simulink model "CCModel_71"  (R2024a)
settings: Solver=ode3  StartTime=0.0  StopTime=100  FixedStep=0.001  RelTol=1e-3  EnableMultiTasking=on
undefined symbols (not defined in the file or in its folder): DiscIntNeverNeededParam, Hecate_desVel1, Hecate_desVel2, Hecate_desVel3, Hecate_horShift, Hecate_period, Hecate_slope, Hecate_Transition1, Hecate_Transition2, Hecate_verShift, i, PME_qb, qb_map, RPM_qb, V
libraries: simulink x46
(part 5 of 11)

== system CCModel_71/Cruise Control/Version 6.4/Sigmoid ==
  note: This whole part is just to eliminate weird cancellation errors that were happening
  U1 : Inport
  U2 : Inport  Port=2
  Change_time : Inport  Port=3
  Abs : Abs  SaturateOnIntegerOverflow=off
  Abs2 : Abs  SaturateOnIntegerOverflow=off
  Add Constant : Bias  Bias=1  SaturateOnIntegerOverflow=off
  Add Constant2 : Bias  Bias=1  SaturateOnIntegerOverflow=off
  Add Constant3 : Bias  Bias=1  SaturateOnIntegerOverflow=off
  Add3 : Sum
  Add4 : Sum  Inputs=+-
  Add5 : Sum
  Clock1 : Clock
  Constant : Constant
  Constant3 : Constant
  Divide : Product  Inputs=/*
  Divide1 : Product  Inputs=**
  Divide4 : Product  Inputs=*/
  Divide5 : Product  Inputs=**
  Divide6 : Product  Inputs=**
  Divide8 : Product  Inputs=*/
  Gain : Gain  Gain=1/2
  Gain1 : Gain  Gain=2
  Gain2 : Gain  Gain=1000
  Gain3 : Gain  Gain=0.001
  Gain5 : Gain  Gain=1/2
  K : Constant
  Power{,3..5} (4 alike) : Math  Operator=pow
  Reciprocal : Product  Inputs=/
  Reciprocal2 : Product  Inputs=/
  Round1 : Rounding  Operator=round
  Scope : Scope  NumInputPorts=3
  Subtract : Sum  Inputs=+-
  Subtract1 : Sum  Inputs=+-
  Subtract2 : Sum  Inputs=+-
  Sum1 : Sum  Inputs=|-+
  h : Constant  Value=4
  u_out : Outport
  wires:
  Add5/1 -> Scope/1, u_out/1
  h/1 -> Abs2/1, Divide8/1, Subtract/2
  Add3/1 -> Divide6/2
  Add4/1 -> Divide5/1
  Constant3/1 -> Add3/2, Add4/1
  Power5/1 -> Divide4/2
  Reciprocal2/1 -> Power5/2
  K/1 -> Power4/2, Reciprocal2/1, Reciprocal/1, Power/2
  Gain5/1 -> Divide6/1
  Change_time/1 -> Sum1/1
  Abs/1 -> Power4/1
  Clock1/1 -> Sum1/2
  Gain3/1 -> Subtract/1
  U2/1 -> Gain5/1, Scope/2, Divide1/1
  Round1/1 -> Gain3/1
  Power4/1 -> Add Constant/1
  Gain2/1 -> Round1/1
  Add Constant/1 -> Power5/1
  Subtract/1 -> Divide4/1, Abs/1
  U1/1 -> Subtract2/1, Scope/3
  Divide6/1 -> Add5/1
  Sum1/1 -> Gain2/1  "Elapsed Time"
  Divide4/1 -> Add3/1, Add4/2
  Abs2/1 -> Power/1
  Power/1 -> Add Constant2/1
  Add Constant2/1 -> Power3/1
  Reciprocal/1 -> Power3/2
  Power3/1 -> Divide8/2
  Divide8/1 -> Add Constant3/1
  Add Constant3/1 -> Gain/1
  Constant/1 -> Subtract1/1
  Gain/1 -> Gain1/1, Subtract1/2  "P"
  Subtract1/1 -> Divide1/2
  Divide1/1 -> Subtract2/2
  Subtract2/1 -> Divide/2
  Gain1/1 -> Divide/1
  Divide/1 -> Divide5/2
  Divide5/1 -> Add5/2

== system CCModel_71/Cruise Control/Version 6.4/Switches ==
  U : Inport
  Throttle_In : Inport  Port=2
  Brake_In : Inport  Port=3
  Brake_Switch1 : Switch  Criteria=u2 > Threshold  SaturateOnIntegerOverflow=off  InputSameDT=off
  Brake_Switch3 : Switch  Criteria=u2 > Threshold  Threshold=5  SaturateOnIntegerOverflow=off  InputSameDT=off
  Constant : Constant  Value=0
  Constant3 : Constant  Value=0
  Constant4 : Constant  Value=10
  Constant5 : Constant  Value=10
  Gain11 : Gain  Gain=0.9
  Gain13 : Gain  Gain=-1
  Gain8 : Gain  Gain=0.9
  Max1 : MinMax  Function=max  Inputs=2
  Plus2 : Sum
  Plus3 : Sum
  Polynomial : Polyval  Coefs=[-0.011, -0.12,0.9,10]
  Polynomial1 : Polyval  Coefs=[-0.011, -0.12,0.9,10]
  Ramp1 : simulink/Sources/Ramp  slope=1  start=0  InitialOutput=-100
  Saturation1 : Saturate  UpperLimit=100  LowerLimit=-100
  Scope1 : Scope  NumInputPorts=3
  Switch : Switch  Criteria=u2 > Threshold  Threshold=-10  SaturateOnIntegerOverflow=off  InputSameDT=off
  Switch1 : Switch  Criteria=u2 > Threshold  Threshold=10  SaturateOnIntegerOverflow=off  InputSameDT=off
  Throttle_Switch1 : Switch  Criteria=u2 > Threshold  SaturateOnIntegerOverflow=off  InputSameDT=off
  Throttle_Switch3 : Switch  Criteria=u2 > Threshold  Threshold=5  SaturateOnIntegerOverflow=off  InputSameDT=off
  Throttle : Outport
  Brake : Outport  Port=2
  wires:
  Plus2/1 -> Throttle_Switch1/1
  Gain8/1 -> Plus2/1
  Constant4/1 -> Plus2/2
  Gain13/1 -> Polynomial1/1, Gain11/1, Brake_Switch1/2
  Constant5/1 -> Plus3/2
  Brake_Switch1/1 -> Brake_Switch3/3  "Brake"
  Throttle_Switch1/1 -> Throttle_Switch3/3  "Throttle"
  Gain11/1 -> Plus3/1
  Brake_Switch3/1 -> Scope1/3, Brake/1
  Brake_In/1 -> Brake_Switch3/1, Max1/2
  Switch/1 -> Throttle_Switch1/3
  Throttle_In/1 -> Throttle_Switch3/1, Max1/1
  Saturation1/1 -> Switch/2, Switch1/2, Gain13/1, Gain8/1, Throttle_Switch1/2, Scope1/1, Polynomial/1
  Polynomial/1 -> Switch/1
  Polynomial1/1 -> Switch1/3
  Constant/1 -> Switch/3
  Switch1/1 -> Brake_Switch1/3
  Constant3/1 -> Switch1/1
  Throttle_Switch3/1 -> Scope1/2, Throttle/1
  Max1/1 -> Throttle_Switch3/2, Brake_Switch3/2
  Plus3/1 -> Brake_Switch1/1
  U/1 -> Saturation1/1

== system CCModel_71/Cruise Control/Version 6.5/Apply_Grade ==
  note: This has not been implemented but may be helpful
  note: +(2/5)|P|
  note: x is u, which is linear and g is grade which is sigmoided
  U_in : Inport
  Grade : Inport  Port=2
  Add : Sum
  Add Constant : Bias  Bias=1  SaturateOnIntegerOverflow=off
  Divide : Product  Inputs=*/
  Gain : Gain  Gain=0.8
  Gain1 : Gain  Gain=0.25
  Scope : Scope  NumInputPorts=2
  Sqrt : Sqrt
  Square : Math  Operator=square
  U_Out : Outport
  wires:
  U_in/1 -> Scope/1, Gain/1
  Square/1 -> Add Constant/1
  Add Constant/1 -> Sqrt/1
  Grade/1 -> Gain1/1, Square/1
  Gain1/1 -> Divide/1
  Sqrt/1 -> Divide/2
  Divide/1 -> Add/2
  Gain/1 -> Add/1
  Add/1 -> Scope/2, U_Out/1

== system CCModel_71/Cruise Control/Version 6.5/Detect Change ==
  note: This subsystem detects either a change in the reference velocity, or the driver releasing one of the pedals. It outputs the time of the change, the value of u just before the change, and a boolean "hasChanged" value
  desired_velocity : Inport
  throttle_const : Inport  Port=2
  brake_const : Inport  Port=3
  Smoothed u : Inport  Port=4
  (False) : Constant  Value=0
  (True) : Constant
  AND : Logic  IconShape=distinctive  AllPortsSameDT=off  OutDataTypeStr=boolean
  Clock : Clock
  Constant : Constant  Value=0.01
  Delay : Delay  DelayLength=1
  Delay1 : Delay  DelayLength=1
  Detect Change : simulink/Logic and Bit Operations/Detect Change  vinit=0  OutDataTypeStr=boolean
  Detect Change1 : simulink/Logic and Bit Operations/Detect Change  vinit=0  OutDataTypeStr=boolean
  Max : MinMax  Function=max  Inputs=2
  Max1 : MinMax  Function=max  Inputs=2
  OR : Logic  Operator=OR  IconShape=distinctive  AllPortsSameDT=off  OutDataTypeStr=boolean
  Pedal_threshold : Constant
  Scope : Scope
  Subtract : Sum  Inputs=+-
  Switch : Switch  Criteria=u2 > Threshold  SaturateOnIntegerOverflow=off  InputSameDT=off
  Switch1 : Switch  Criteria=u2 > Threshold  SaturateOnIntegerOverflow=off  InputSameDT=off
  Switch2 : Switch  Criteria=u2 > Threshold  SaturateOnIntegerOverflow=off  InputSameDT=off
  Change_time : Outport
  Old u : Outport  Port=2
  hasChanged : Outport  Port=3
  wires:
  desired_velocity/1 -> Detect Change/1
  Detect Change/1 -> OR/1
  OR/1 -> Switch/2, Switch2/2, hasChanged/1
  Switch1/1 -> Detect Change1/1, Delay1/1
  AND/1 -> OR/2
  Clock/1 -> Switch/1
  Max/1 -> Subtract/1
  (True)/1 -> Switch1/1
  brake_const/1 -> Max/2
  Pedal_threshold/1 -> Subtract/2
  Subtract/1 -> Switch1/2
  (False)/1 -> Switch1/3
  throttle_const/1 -> Max/1
  Switch2/1 -> Switch2/3, Max1/1
  Delay/1 -> Switch2/1
  Switch/1 -> Switch/3, Scope/1, Change_time/1
  Smoothed u/1 -> Delay/1
  Detect Change1/1 -> AND/2
  Delay1/1 -> AND/1
  Constant/1 -> Max1/2
  Max1/1 -> Old u/1

== system CCModel_71/Cruise Control/Version 6.5/PID Controller ==
  note: Typical PID controller, outputs a value between -100 and 100
  error : Inport
  Grade : Inport  Port=2
  Add : Sum
  Add1 : Sum
  Derivative : Derivative
  GKi : Gain  Gain=0
  GKp : Gain  Gain=0
  Integrator : Integrator
  Integrator1 : Integrator
  Kd : Gain  Gain=0.1
  Ki : Gain  Gain=0.03
  Kp : Gain  Gain=4
  Saturation : Saturate  UpperLimit=100  LowerLimit=-100
  Scope1 : Scope  NumInputPorts=3
  Sum : Sum  Inputs=+++
  u : Outport
  wires:
  Integrator/1 -> Ki/1
  error/1 -> Integrator/1, Kp/1, Derivative/1  "D"
  Kp/1 -> Scope1/1, Sum/2  "P"
  Ki/1 -> Sum/1, Scope1/2  "I"
  Saturation/1 -> u/1
  Derivative/1 -> Kd/1
  Kd/1 -> Scope1/3, Sum/3  "D"
  Sum/1 -> Add1/1
  Add1/1 -> Saturation/1
  Grade/1 -> Integrator1/1, GKp/1
  Integrator1/1 -> GKi/1
  GKi/1 -> Add/1
  GKp/1 -> Add/2
  Add/1 -> Add1/2

== system CCModel_71/Cruise Control/Version 6.5/Sigmoid ==
  note: This whole part is just to eliminate weird cancellation errors that were happening
  U1 : Inport
  U2 : Inport  Port=2
  Change_time : Inport  Port=3
  Abs : Abs  SaturateOnIntegerOverflow=off
  Abs2 : Abs  SaturateOnIntegerOverflow=off
  Add Constant : Bias  Bias=1  SaturateOnIntegerOverflow=off
  Add Constant2 : Bias  Bias=1  SaturateOnIntegerOverflow=off
  Add Constant3 : Bias  Bias=1  SaturateOnIntegerOverflow=off
  Add3 : Sum
  Add4 : Sum  Inputs=+-
  Add5 : Sum
  Clock1 : Clock
  Constant : Constant
  Constant3 : Constant
  Divide : Product  Inputs=/*
  Divide1 : Product  Inputs=**
  Divide4 : Product  Inputs=*/
  Divide5 : Product  Inputs=**
  Divide6 : Product  Inputs=**
  Divide8 : Product  Inputs=*/
  Gain : Gain  Gain=1/2
  Gain1 : Gain  Gain=2
  Gain2 : Gain  Gain=1000
  Gain3 : Gain  Gain=0.001
  Gain5 : Gain  Gain=1/2
  K : Constant  Value=1.5
  Power{,3..5} (4 alike) : Math  Operator=pow
  Reciprocal : Product  Inputs=/
  Reciprocal2 : Product  Inputs=/
  Round1 : Rounding  Operator=round
  Scope : Scope  NumInputPorts=3
  Subtract : Sum  Inputs=+-
  Subtract1 : Sum  Inputs=+-
  Subtract2 : Sum  Inputs=+-
  Sum1 : Sum  Inputs=|-+
  h : Constant  Value=4
  u_out : Outport
  wires:
  Add5/1 -> Scope/1, u_out/1
  h/1 -> Abs2/1, Divide8/1, Subtract/2
  Add3/1 -> Divide6/2
  Add4/1 -> Divide5/1
  Constant3/1 -> Add3/2, Add4/1
  Power5/1 -> Divide4/2
  Reciprocal2/1 -> Power5/2
  K/1 -> Power4/2, Reciprocal2/1, Reciprocal/1, Power/2
  Gain5/1 -> Divide6/1
  Change_time/1 -> Sum1/1
  Abs/1 -> Power4/1
  Clock1/1 -> Sum1/2
  Gain3/1 -> Subtract/1
  U2/1 -> Gain5/1, Scope/2, Divide1/1
  Round1/1 -> Gain3/1
  Power4/1 -> Add Constant/1
  Gain2/1 -> Round1/1
  Add Constant/1 -> Power5/1
  Subtract/1 -> Divide4/1, Abs/1
  U1/1 -> Subtract2/1, Scope/3
  Divide6/1 -> Add5/1
  Sum1/1 -> Gain2/1  "Elapsed Time"
  Divide4/1 -> Add3/1, Add4/2
  Abs2/1 -> Power/1
  Power/1 -> Add Constant2/1
  Add Constant2/1 -> Power3/1
  Reciprocal/1 -> Power3/2
  Power3/1 -> Divide8/2
  Divide8/1 -> Add Constant3/1
  Add Constant3/1 -> Gain/1
  Constant/1 -> Subtract1/1
  Gain/1 -> Gain1/1, Subtract1/2  "P"
  Subtract1/1 -> Divide1/2
  Divide1/1 -> Subtract2/2
  Subtract2/1 -> Divide/2
  Gain1/1 -> Divide/1
  Divide/1 -> Divide5/2
  Divide5/1 -> Add5/2

== system CCModel_71/Cruise Control/Version 6.5/Switches ==
  U : Inport
  Throttle_In : Inport  Port=2
  Brake_In : Inport  Port=3
  Brake_Switch1 : Switch  Criteria=u2 > Threshold  SaturateOnIntegerOverflow=off  InputSameDT=off
  Brake_Switch3 : Switch  Criteria=u2 > Threshold  Threshold=5  SaturateOnIntegerOverflow=off  InputSameDT=off
  Constant : Constant  Value=0
  Constant1 : Constant  Value=0
  Gain13 : Gain  Gain=-1
  Max1 : MinMax  Function=max  Inputs=2
  Polynomial : Polyval  Coefs=[-0.01,0.2,0,0]
  Polynomial1 : Polyval  Coefs=[-0.01,0.2,0,0]
  Ramp1 : simulink/Sources/Ramp  slope=5  start=0  InitialOutput=-100
  Saturation1 : Saturate  UpperLimit=100  LowerLimit=-100
  Scope1 : Scope  NumInputPorts=3
  Switch : Switch  Criteria=u2 > Threshold  Threshold=10  SaturateOnIntegerOverflow=off  InputSameDT=off
  Switch1 : Switch  Criteria=u2 > Threshold  Threshold=10  SaturateOnIntegerOverflow=off  InputSameDT=off
  Throttle_Switch1 : Switch  Criteria=u2 > Threshold  SaturateOnIntegerOverflow=off  InputSameDT=off
  Throttle_Switch3 : Switch  Criteria=u2 > Threshold  Threshold=5  SaturateOnIntegerOverflow=off  InputSameDT=off
  Throttle : Outport
  Brake : Outport  Port=2
  wires:
  Gain13/1 -> Polynomial1/1, Switch1/2, Switch1/1, Brake_Switch1/2
  Brake_Switch1/1 -> Brake_Switch3/3  "Brake"
  Throttle_Switch1/1 -> Throttle_Switch3/3  "Throttle"
  Brake_Switch3/1 -> Scope1/3, Brake/1
  Brake_In/1 -> Brake_Switch3/1, Max1/2
  Throttle_In/1 -> Throttle_Switch3/1, Max1/1
  Polynomial1/1 -> Switch1/3
  Throttle_Switch3/1 -> Scope1/2, Throttle/1
  Constant1/1 -> Brake_Switch1/3, Throttle_Switch1/3
  Switch/1 -> Throttle_Switch1/1
  Polynomial/1 -> Switch/3
  Switch1/1 -> Brake_Switch1/1
  Saturation1/1 -> Gain13/1, Switch/1, Switch/2, Scope1/1, Polynomial/1, Throttle_Switch1/2
  U/1 -> Saturation1/1
  Max1/1 -> Throttle_Switch3/2, Brake_Switch3/2

== system CCModel_71/Cruise Control/Version 6.6/Apply_Grade ==
  note: This has not been implemented but may be helpful
  note: +(2/5)|P|
  note: x is u, which is linear and g is grade which is sigmoided
  U_in : Inport
  Grade : Inport  Port=2
  Add : Sum
  Add Constant : Bias  Bias=1  SaturateOnIntegerOverflow=off
  Divide : Product  Inputs=*/
  Gain : Gain  Gain=0.8
  Gain1 : Gain  Gain=0.25
  Scope : Scope  NumInputPorts=2
  Sqrt : Sqrt
  Square : Math  Operator=square
  U_Out : Outport
  wires:
  U_in/1 -> Scope/1, Gain/1
  Square/1 -> Add Constant/1
  Add Constant/1 -> Sqrt/1
  Grade/1 -> Gain1/1, Square/1
  Gain1/1 -> Divide/1
  Sqrt/1 -> Divide/2
  Divide/1 -> Add/2
  Gain/1 -> Add/1
  Add/1 -> Scope/2, U_Out/1

== system CCModel_71/Cruise Control/Version 6.6/Detect Change ==
  note: This subsystem detects either a change in the reference velocity, or the driver releasing one of the pedals. It outputs the time of the change, the value of u just before the change, and a boolean "hasChanged" value
  desired_velocity : Inport
  throttle_const : Inport  Port=2
  brake_const : Inport  Port=3
  Smoothed u : Inport  Port=4
  (False) : Constant  Value=0
  (True) : Constant
  AND : Logic  IconShape=distinctive  AllPortsSameDT=off  OutDataTypeStr=boolean
  Clock : Clock
  Constant : Constant  Value=0.01
  Delay : Delay  DelayLength=1
  Delay1 : Delay  DelayLength=1
  Detect Change : simulink/Logic and Bit Operations/Detect Change  vinit=0  OutDataTypeStr=boolean
  Detect Change1 : simulink/Logic and Bit Operations/Detect Change  vinit=0  OutDataTypeStr=boolean
  Max : MinMax  Function=max  Inputs=2
  Max1 : MinMax  Function=max  Inputs=2
  OR : Logic  Operator=OR  IconShape=distinctive  AllPortsSameDT=off  OutDataTypeStr=boolean
  Pedal_threshold : Constant
  Scope : Scope
  Subtract : Sum  Inputs=+-
  Switch : Switch  Criteria=u2 > Threshold  SaturateOnIntegerOverflow=off  InputSameDT=off
  Switch1 : Switch  Criteria=u2 > Threshold  SaturateOnIntegerOverflow=off  InputSameDT=off
  Switch2 : Switch  Criteria=u2 > Threshold  SaturateOnIntegerOverflow=off  InputSameDT=off
  Change_time : Outport
  Old u : Outport  Port=2
  hasChanged : Outport  Port=3
  wires:
  desired_velocity/1 -> Detect Change/1
  Detect Change/1 -> OR/1
  OR/1 -> Switch/2, Switch2/2, hasChanged/1
  Switch1/1 -> Detect Change1/1, Delay1/1
  AND/1 -> OR/2
  Clock/1 -> Switch/1
  Max/1 -> Subtract/1
  (True)/1 -> Switch1/1
  brake_const/1 -> Max/2
  Pedal_threshold/1 -> Subtract/2
  Subtract/1 -> Switch1/2
  (False)/1 -> Switch1/3
  throttle_const/1 -> Max/1
  Switch2/1 -> Switch2/3, Max1/1
  Delay/1 -> Switch2/1
  Switch/1 -> Switch/3, Scope/1, Change_time/1
  Smoothed u/1 -> Delay/1
  Detect Change1/1 -> AND/2
  Delay1/1 -> AND/1
  Constant/1 -> Max1/2
  Max1/1 -> Old u/1

== system CCModel_71/Cruise Control/Version 6.6/PID Controller ==
  note: Typical PID controller, outputs a value between -100 and 100
  error : Inport
  Grade : Inport  Port=2
  Add : Sum
  Add1 : Sum
  Derivative : Derivative
  GKi : Gain  Gain=0
  GKp : Gain  Gain=0
  Integrator : Integrator
  Integrator1 : Integrator
  Kd : Gain  Gain=0.1
  Ki : Gain  Gain=0.03
  Kp : Gain  Gain=3
  Saturation : Saturate  Commented=through  UpperLimit=100  LowerLimit=-100
  Scope1 : Scope  NumInputPorts=3
  Sum : Sum  Inputs=+++
  u : Outport
  wires:
  Integrator/1 -> Ki/1
  error/1 -> Integrator/1, Kp/1, Derivative/1  "D"
  Kp/1 -> Scope1/1, Sum/2  "P"
  Ki/1 -> Sum/1, Scope1/2  "I"
  Saturation/1 -> u/1
  Derivative/1 -> Kd/1
  Kd/1 -> Scope1/3, Sum/3  "D"
  Sum/1 -> Add1/1
  Add1/1 -> Saturation/1
  Grade/1 -> Integrator1/1, GKp/1
  Integrator1/1 -> GKi/1
  GKi/1 -> Add/1
  GKp/1 -> Add/2
  Add/1 -> Add1/2

== system CCModel_71/Cruise Control/Version 6.6/Sigmoid ==
  note: This whole part is just to eliminate weird cancellation errors that were happening
  U1 : Inport
  U2 : Inport  Port=2
  Change_time : Inport  Port=3
  Abs : Abs  SaturateOnIntegerOverflow=off
  Abs2 : Abs  SaturateOnIntegerOverflow=off
  Add Constant : Bias  Bias=1  SaturateOnIntegerOverflow=off
  Add Constant2 : Bias  Bias=1  SaturateOnIntegerOverflow=off
  Add Constant3 : Bias  Bias=1  SaturateOnIntegerOverflow=off
  Add3 : Sum
  Add4 : Sum  Inputs=+-
  Add5 : Sum
  Clock1 : Clock
  Constant : Constant
  Constant3 : Constant
  Divide : Product  Inputs=/*
  Divide1 : Product  Inputs=**
  Divide4 : Product  Inputs=*/
  Divide5 : Product  Inputs=**
  Divide6 : Product  Inputs=**
  Divide8 : Product  Inputs=*/
  Gain : Gain  Gain=1/2
  Gain1 : Gain  Gain=2
  Gain2 : Gain  Gain=1000
  Gain3 : Gain  Gain=0.001
  Gain5 : Gain  Gain=1/2
  K : Constant  Value=1.5
  Power{,3..5} (4 alike) : Math  Operator=pow
  Reciprocal : Product  Inputs=/
  Reciprocal2 : Product  Inputs=/
  Round1 : Rounding  Operator=round
  Saturation : Saturate  UpperLimit=100  LowerLimit=-100
  Scope : Scope  NumInputPorts=3
  Subtract : Sum  Inputs=+-
  Subtract1 : Sum  Inputs=+-
  Subtract2 : Sum  Inputs=+-
  Sum1 : Sum  Inputs=|-+
  h : Constant  Value=4
  u_out : Outport
  wires:
  Add5/1 -> Scope/1, Saturation/1
  h/1 -> Abs2/1, Divide8/1, Subtract/2
  Add3/1 -> Divide6/2
  Add4/1 -> Divide5/1
  Constant3/1 -> Add3/2, Add4/1
  Power5/1 -> Divide4/2
  Reciprocal2/1 -> Power5/2
  K/1 -> Power4/2, Reciprocal2/1, Reciprocal/1, Power/2
  Gain5/1 -> Divide6/1
  Change_time/1 -> Sum1/1
  Abs/1 -> Power4/1
  Clock1/1 -> Sum1/2
  Gain3/1 -> Subtract/1
  U2/1 -> Gain5/1, Scope/2, Divide1/1
  Round1/1 -> Gain3/1
  Power4/1 -> Add Constant/1
  Gain2/1 -> Round1/1
  Add Constant/1 -> Power5/1
  Subtract/1 -> Divide4/1, Abs/1
  U1/1 -> Subtract2/1, Scope/3
  Divide6/1 -> Add5/1
  Sum1/1 -> Gain2/1  "Elapsed Time"
  Divide4/1 -> Add3/1, Add4/2
  Abs2/1 -> Power/1
  Power/1 -> Add Constant2/1
  Add Constant2/1 -> Power3/1
  Reciprocal/1 -> Power3/2
  Power3/1 -> Divide8/2
  Divide8/1 -> Add Constant3/1
  Add Constant3/1 -> Gain/1
  Constant/1 -> Subtract1/1
  Gain/1 -> Gain1/1, Subtract1/2  "P"
  Subtract1/1 -> Divide1/2
  Divide1/1 -> Subtract2/2
  Subtract2/1 -> Divide/2
  Gain1/1 -> Divide/1
  Divide/1 -> Divide5/2
  Divide5/1 -> Add5/2
  Saturation/1 -> u_out/1

== system CCModel_71/Cruise Control/Version 6.6/Switches ==
  U : Inport
  Throttle_In : Inport  Port=2
  Brake_In : Inport  Port=3
  Brake_Switch1 : Switch  Criteria=u2 > Threshold  SaturateOnIntegerOverflow=off  InputSameDT=off
  Brake_Switch3 : Switch  Criteria=u2 > Threshold  Threshold=5  SaturateOnIntegerOverflow=off  InputSameDT=off
  Constant : Constant  Value=0
  Constant1 : Constant  Value=0
  Gain13 : Gain  Gain=-1
  Max1 : MinMax  Function=max  Inputs=2
  Polynomial : Polyval  Coefs=[-0.01,0.2,0,0]
  Polynomial1 : Polyval  Coefs=[-0.01,0.2,0,0]
  Ramp1 : simulink/Sources/Ramp  slope=5  start=0  InitialOutput=-100
  Saturation1 : Saturate  UpperLimit=100  LowerLimit=-100
  Scope1 : Scope  NumInputPorts=3
  Switch : Switch  Criteria=u2 > Threshold  Threshold=10  SaturateOnIntegerOverflow=off  InputSameDT=off
  Switch1 : Switch  Criteria=u2 > Threshold  Threshold=10  SaturateOnIntegerOverflow=off  InputSameDT=off
  Throttle_Switch1 : Switch  Criteria=u2 > Threshold  SaturateOnIntegerOverflow=off  InputSameDT=off
  Throttle_Switch3 : Switch  Criteria=u2 > Threshold  Threshold=5  SaturateOnIntegerOverflow=off  InputSameDT=off
  Throttle : Outport
  Brake : Outport  Port=2
  wires:
  Gain13/1 -> Polynomial1/1, Switch1/2, Switch1/1, Brake_Switch1/2
  Brake_Switch1/1 -> Brake_Switch3/3  "Brake"
  Throttle_Switch1/1 -> Throttle_Switch3/3  "Throttle"
  Brake_Switch3/1 -> Scope1/3, Brake/1
  Brake_In/1 -> Brake_Switch3/1, Max1/2
  Throttle_In/1 -> Throttle_Switch3/1, Max1/1
  Polynomial1/1 -> Switch1/3
  Throttle_Switch3/1 -> Scope1/2, Throttle/1
  Constant1/1 -> Brake_Switch1/3, Throttle_Switch1/3
  Switch/1 -> Throttle_Switch1/1
  Polynomial/1 -> Switch/3
  Switch1/1 -> Brake_Switch1/1
  Saturation1/1 -> Gain13/1, Switch/1, Switch/2, Scope1/1, Polynomial/1, Throttle_Switch1/2
  U/1 -> Saturation1/1
  Max1/1 -> Throttle_Switch3/2, Brake_Switch3/2

== system CCModel_71/Cruise Control/Version 7.0/Apply_Grade ==
  note: This has not been implemented but may be helpful
  note: +(2/5)|P|
  note: x is u, which is linear and g is grade which is sigmoided
  U_in : Inport
  Grade : Inport  Port=2
  Add : Sum
  Add Constant : Bias  Bias=1  SaturateOnIntegerOverflow=off
  Divide : Product  Inputs=*/
  Gain : Gain  Gain=0.8
  Gain1 : Gain  Gain=0.25
  Scope : Scope  NumInputPorts=2
  Sqrt : Sqrt
  Square : Math  Operator=square
  U_Out : Outport
  wires:
  U_in/1 -> Scope/1, Gain/1
  Square/1 -> Add Constant/1
  Add Constant/1 -> Sqrt/1
  Grade/1 -> Gain1/1, Square/1
  Gain1/1 -> Divide/1
  Sqrt/1 -> Divide/2
  Divide/1 -> Add/2
  Gain/1 -> Add/1
  Add/1 -> Scope/2, U_Out/1

== system CCModel_71/Cruise Control/Version 7.0/Detect Change ==
  note: This subsystem detects either a change in the reference velocity, or the driver releasing one of the pedals. It outputs the time of the change, the value of u just before the change, and a boolean "hasChanged" value
  desired_velocity : Inport
  throttle_const : Inport  Port=2
  brake_const : Inport  Port=3
  Smoothed u : Inport  Port=4
  (False) : Constant  Value=0
  (True) : Constant
  AND : Logic  IconShape=distinctive  AllPortsSameDT=off  OutDataTypeStr=boolean
  Clock : Clock
  Constant : Constant  Value=0.01
  Delay : Delay  DelayLength=1
  Delay1 : Delay  DelayLength=1
  Detect Change : simulink/Logic and Bit Operations/Detect Change  vinit=0  OutDataTypeStr=boolean
  Detect Change1 : simulink/Logic and Bit Operations/Detect Change  vinit=0  OutDataTypeStr=boolean
  Max : MinMax  Function=max  Inputs=2
  Max1 : MinMax  Function=max  Inputs=2
  OR : Logic  Operator=OR  IconShape=distinctive  AllPortsSameDT=off  OutDataTypeStr=boolean
  Pedal_threshold : Constant
  Scope : Scope
  Subtract : Sum  Inputs=+-
  Switch : Switch  Criteria=u2 > Threshold  SaturateOnIntegerOverflow=off  InputSameDT=off
  Switch1 : Switch  Criteria=u2 > Threshold  SaturateOnIntegerOverflow=off  InputSameDT=off
  Switch2 : Switch  Criteria=u2 > Threshold  SaturateOnIntegerOverflow=off  InputSameDT=off
  Change_time : Outport
  Old u : Outport  Port=2
  hasChanged : Outport  Port=3
  wires:
  desired_velocity/1 -> Detect Change/1
  Detect Change/1 -> OR/1
  OR/1 -> Switch/2, Switch2/2, hasChanged/1
  Switch1/1 -> Detect Change1/1, Delay1/1
  AND/1 -> OR/2
  Clock/1 -> Switch/1
  Max/1 -> Subtract/1
  (True)/1 -> Switch1/1
  brake_const/1 -> Max/2
  Pedal_threshold/1 -> Subtract/2
  Subtract/1 -> Switch1/2
  (False)/1 -> Switch1/3
  throttle_const/1 -> Max/1
  Switch2/1 -> Switch2/3, Max1/1
  Delay/1 -> Switch2/1
  Switch/1 -> Switch/3, Scope/1, Change_time/1
  Smoothed u/1 -> Delay/1
  Detect Change1/1 -> AND/2
  Delay1/1 -> AND/1
  Constant/1 -> Max1/2
  Max1/1 -> Old u/1

== system CCModel_71/Cruise Control/Version 7.0/PID Controller ==
  note: Typical PID controller, outputs a value between -100 and 100
  error : Inport
  Grade : Inport  Port=2
  Add : Sum
  Add1 : Sum
  Derivative : Derivative
  GKi : Gain  Gain=0
  GKp : Gain  Gain=0
  Integrator : Integrator
  Integrator1 : Integrator
  Kd : Gain  Gain=0.1
  Ki : Gain  Gain=0.03
  Kp : Gain  Gain=4
  Saturation : Saturate  Commented=through  UpperLimit=100  LowerLimit=-100
  Scope1 : Scope  NumInputPorts=3
  Sum : Sum  Inputs=+++
  u : Outport
  wires:
  Integrator/1 -> Ki/1
  error/1 -> Integrator/1, Kp/1, Derivative/1  "D"
  Kp/1 -> Scope1/1, Sum/2  "P"
  Ki/1 -> Sum/1, Scope1/2  "I"
  Saturation/1 -> u/1
  Derivative/1 -> Kd/1
  Kd/1 -> Scope1/3, Sum/3  "D"
  Sum/1 -> Add1/1
  Add1/1 -> Saturation/1
  Grade/1 -> Integrator1/1, GKp/1
  Integrator1/1 -> GKi/1
  GKi/1 -> Add/1
  GKp/1 -> Add/2
  Add/1 -> Add1/2

== system CCModel_71/Cruise Control/Version 7.0/Sigmoid ==
  note: This whole part is just to eliminate weird cancellation errors that were happening
  U1 : Inport
  U2 : Inport  Port=2
  Change_time : Inport  Port=3
  Abs : Abs  SaturateOnIntegerOverflow=off
  Abs2 : Abs  SaturateOnIntegerOverflow=off
  Add Constant : Bias  Bias=1  SaturateOnIntegerOverflow=off
  Add Constant2 : Bias  Bias=1  SaturateOnIntegerOverflow=off
  Add Constant3 : Bias  Bias=1  SaturateOnIntegerOverflow=off
  Add3 : Sum
  Add4 : Sum  Inputs=+-
  Add5 : Sum
  Clock1 : Clock
  Constant : Constant
  Constant3 : Constant
  Divide : Product  Inputs=/*
  Divide1 : Product  Inputs=**
  Divide4 : Product  Inputs=*/
  Divide5 : Product  Inputs=**
  Divide6 : Product  Inputs=**
  Divide8 : Product  Inputs=*/
  Gain : Gain  Gain=1/2
  Gain1 : Gain  Gain=2
  Gain2 : Gain  Gain=1000
  Gain3 : Gain  Gain=0.001
  Gain5 : Gain  Gain=1/2
  K : Constant  Value=1.5
  Power{,3..5} (4 alike) : Math  Operator=pow
  Reciprocal : Product  Inputs=/
  Reciprocal2 : Product  Inputs=/
  Round1 : Rounding  Operator=round
  Saturation : Saturate  UpperLimit=100  LowerLimit=-100
  Scope : Scope  NumInputPorts=3
  Subtract : Sum  Inputs=+-
  Subtract1 : Sum  Inputs=+-
  Subtract2 : Sum  Inputs=+-
  Sum1 : Sum  Inputs=|-+
  h : Constant  Value=4
  u_out : Outport
  wires:
  Add5/1 -> Scope/1, Saturation/1
  h/1 -> Abs2/1, Divide8/1, Subtract/2
  Add3/1 -> Divide6/2
  Add4/1 -> Divide5/1
  Constant3/1 -> Add3/2, Add4/1
  Power5/1 -> Divide4/2
  Reciprocal2/1 -> Power5/2
  K/1 -> Power4/2, Reciprocal2/1, Reciprocal/1, Power/2
  Gain5/1 -> Divide6/1
  Change_time/1 -> Sum1/1
  Abs/1 -> Power4/1
  Clock1/1 -> Sum1/2
  Gain3/1 -> Subtract/1
  U2/1 -> Gain5/1, Scope/2, Divide1/1
  Round1/1 -> Gain3/1
  Power4/1 -> Add Constant/1
  Gain2/1 -> Round1/1
  Add Constant/1 -> Power5/1
  Subtract/1 -> Divide4/1, Abs/1
  U1/1 -> Subtract2/1, Scope/3
  Divide6/1 -> Add5/1
  Sum1/1 -> Gain2/1  "Elapsed Time"
  Divide4/1 -> Add3/1, Add4/2
  Abs2/1 -> Power/1
  Power/1 -> Add Constant2/1
  Add Constant2/1 -> Power3/1
  Reciprocal/1 -> Power3/2
  Power3/1 -> Divide8/2
  Divide8/1 -> Add Constant3/1
  Add Constant3/1 -> Gain/1
  Constant/1 -> Subtract1/1
  Gain/1 -> Gain1/1, Subtract1/2  "P"
  Subtract1/1 -> Divide1/2
  Divide1/1 -> Subtract2/2
  Subtract2/1 -> Divide/2
  Gain1/1 -> Divide/1
  Divide/1 -> Divide5/2
  Divide5/1 -> Add5/2
  Saturation/1 -> u_out/1

== system CCModel_71/Cruise Control/Version 7.0/Switches ==
  U : Inport
  Throttle_In : Inport  Port=2
  Brake_In : Inport  Port=3
  Add Constant : Bias  Bias=6  SaturateOnIntegerOverflow=off
  Add Constant1 : Bias  Bias=10  SaturateOnIntegerOverflow=off
  Add Constant2 : Bias  Bias=5  SaturateOnIntegerOverflow=off
  Add Constant3 : Bias  Bias=-10  SaturateOnIntegerOverflow=off
  Brake_Switch1 : Switch  Criteria=u2 > Threshold  Threshold=-10  SaturateOnIntegerOverflow=off  InputSameDT=off
  Brake_Switch2 : Switch  Criteria=u2 > Threshold  Threshold=30  SaturateOnIntegerOverflow=off  InputSameDT=off
  Brake_Switch3 : Switch  Criteria=u2 > Threshold  Threshold=5  SaturateOnIntegerOverflow=off  InputSameDT=off
  Constant : Constant  Value=0
  Constant1 : Constant  Value=0
  Gain : Gain  Gain=-1
  Gain1 : Gain  Gain=pi/40
  Gain2 : Gain  Gain=-5
  Gain3 : Gain  Gain=0.2
  Max1 : MinMax  Function=max  Inputs=2
  Polynomial : Polyval  Coefs=[-0.01,0.2,0,0]
  Polynomial1 : Polyval  Coefs=[0.01,0.2,0,10]
  Ramp1 : simulink/Sources/Ramp  slope=5  start=0  InitialOutput=-100
  Saturation1 : Saturate  UpperLimit=100  LowerLimit=-100
  Scope1 : Scope  NumInputPorts=3
  Sin : Trigonometry
  Switch : Switch  Criteria=u2 > Threshold  Threshold=10  SaturateOnIntegerOverflow=off  InputSameDT=off
  Switch1 : Switch  Criteria=u2 > Threshold  Threshold=-20  SaturateOnIntegerOverflow=off  InputSameDT=off
  Throttle_Switch1 : Switch  Criteria=u2 > Threshold  SaturateOnIntegerOverflow=off  InputSameDT=off
  Throttle_Switch3 : Switch  Criteria=u2 > Threshold  Threshold=5  SaturateOnIntegerOverflow=off  InputSameDT=off
  Throttle : Outport
  Brake : Outport  Port=2
  wires:
  Saturation1/1 -> Brake_Switch2/2, Brake_Switch1/2, Switch1/2, Gain/1, Add Constant3/1, Add Constant1/1, Switch/1, Switch/2, Scope1/1, Polynomial/1, Throttle_Switch1/2
  Throttle_Switch1/1 -> Add Constant/1  "Throttle"
  Brake_Switch3/1 -> Scope1/3, Brake/1
  Brake_In/1 -> Brake_Switch3/1, Max1/2
  Throttle_In/1 -> Throttle_Switch3/1, Max1/1
  Throttle_Switch3/1 -> Scope1/2, Throttle/1
  Constant1/1 -> Throttle_Switch1/3, Brake_Switch2/1
  Switch/1 -> Throttle_Switch1/1
  Polynomial/1 -> Switch/3
  Max1/1 -> Throttle_Switch3/2, Brake_Switch3/2
  Add Constant/1 -> Throttle_Switch3/3
  Add Constant1/1 -> Polynomial1/1
  Gain/1 -> Switch1/3
  Polynomial1/1 -> Switch1/1
  Switch1/1 -> Brake_Switch1/3
  Gain1/1 -> Sin/1
  Sin/1 -> Gain2/1
  Gain2/1 -> Add Constant2/1
  Add Constant2/1 -> Brake_Switch1/1
  Brake_Switch2/1 -> Gain3/1  "Brake"
  Brake_Switch1/1 -> Brake_Switch2/3  "Brake"
  U/1 -> Saturation1/1
  Add Constant3/1 -> Gain1/1
  Gain3/1 -> Brake_Switch3/3

== system CCModel_71/Cruise Control/Version 7.1/Apply_Grade ==
  note: This has not been implemented but may be helpful
  note: +(2/5)|P|
  note: x is u, which is linear and g is grade which is sigmoided
  U_in : Inport
  Grade : Inport  Port=2
  Add : Sum
  Add Constant : Bias  Bias=1  SaturateOnIntegerOverflow=off
  Divide : Product  Inputs=*/
  Gain : Gain  Gain=0.8
  Gain1 : Gain  Gain=0.25
  Scope : Scope  NumInputPorts=2
  Sqrt : Sqrt
  Square : Math  Operator=square
  U_Out : Outport
  wires:
  U_in/1 -> Scope/1, Gain/1
  Square/1 -> Add Constant/1
  Add Constant/1 -> Sqrt/1
  Grade/1 -> Gain1/1, Square/1
  Gain1/1 -> Divide/1
  Sqrt/1 -> Divide/2
  Divide/1 -> Add/2
  Gain/1 -> Add/1
  Add/1 -> Scope/2, U_Out/1

== system CCModel_71/Cruise Control/Version 7.1/Detect Change ==
  note: This subsystem detects either a change in the reference velocity, or the driver releasing one of the pedals. It outputs the time of the change, the value of u just before the change, and a boolean "hasChanged" value
  desired_velocity : Inport
  throttle_const : Inport  Port=2
  brake_const : Inport  Port=3
  Smoothed u : Inport  Port=4
  (False) : Constant  Value=0
  (True) : Constant
  AND : Logic  IconShape=distinctive  AllPortsSameDT=off  OutDataTypeStr=boolean
  Clock : Clock
  Constant : Constant  Value=0.01
  Delay : Delay  DelayLength=1
  Delay1 : Delay  DelayLength=1
  Detect Change : simulink/Logic and Bit Operations/Detect Change  vinit=0  OutDataTypeStr=boolean
  Detect Change1 : simulink/Logic and Bit Operations/Detect Change  vinit=0  OutDataTypeStr=boolean
  Max : MinMax  Function=max  Inputs=2
  Max1 : MinMax  Function=max  Inputs=2
  OR : Logic  Operator=OR  IconShape=distinctive  AllPortsSameDT=off  OutDataTypeStr=boolean
  Pedal_threshold : Constant
  Scope : Scope
  Subtract : Sum  Inputs=+-
  Switch : Switch  Criteria=u2 > Threshold  SaturateOnIntegerOverflow=off  InputSameDT=off
  Switch1 : Switch  Criteria=u2 > Threshold  SaturateOnIntegerOverflow=off  InputSameDT=off
  Switch2 : Switch  Criteria=u2 > Threshold  SaturateOnIntegerOverflow=off  InputSameDT=off
  Change_time : Outport
  Old u : Outport  Port=2
  hasChanged : Outport  Port=3
  wires:
  desired_velocity/1 -> Detect Change/1
  Detect Change/1 -> OR/1
  OR/1 -> Switch/2, Switch2/2, hasChanged/1
  Switch1/1 -> Detect Change1/1, Delay1/1
  AND/1 -> OR/2
  Clock/1 -> Switch/1
  Max/1 -> Subtract/1
  (True)/1 -> Switch1/1
  brake_const/1 -> Max/2
  Pedal_threshold/1 -> Subtract/2
  Subtract/1 -> Switch1/2
  (False)/1 -> Switch1/3
  throttle_const/1 -> Max/1
  Switch2/1 -> Switch2/3, Max1/1
  Delay/1 -> Switch2/1
  Switch/1 -> Switch/3, Scope/1, Change_time/1
  Smoothed u/1 -> Delay/1
  Detect Change1/1 -> AND/2
  Delay1/1 -> AND/1
  Constant/1 -> Max1/2
  Max1/1 -> Old u/1

== system CCModel_71/Cruise Control/Version 7.1/PID Controller ==
  note: Typical PID controller, outputs a value between -100 and 100
  error : Inport
  Grade : Inport  Port=2
  Add : Sum
  Add1 : Sum
  Derivative : Derivative
  GKi : Gain  Gain=0
  GKp : Gain  Gain=0
  Integrator : Integrator
  Integrator1 : Integrator
  Kd : Gain  Gain=0.1
  Ki : Gain  Gain=0.03
  Kp : Gain  Gain=4
  Saturation : Saturate  Commented=through  UpperLimit=100  LowerLimit=-100
  Scope1 : Scope  NumInputPorts=3
  Sum : Sum  Inputs=+++
  u : Outport
  wires:
  Integrator/1 -> Ki/1
  error/1 -> Integrator/1, Kp/1, Derivative/1  "D"
  Kp/1 -> Scope1/1, Sum/2  "P"
  Ki/1 -> Sum/1, Scope1/2  "I"
  Saturation/1 -> u/1
  Derivative/1 -> Kd/1
  Kd/1 -> Scope1/3, Sum/3  "D"
  Sum/1 -> Add1/1
  Add1/1 -> Saturation/1
  Grade/1 -> Integrator1/1, GKp/1
  Integrator1/1 -> GKi/1
  GKi/1 -> Add/1
  GKp/1 -> Add/2
  Add/1 -> Add1/2

== system CCModel_71/Cruise Control/Version 7.1/Sigmoid ==
  note: This whole part is just to eliminate weird cancellation errors that were happening
  U1 : Inport
  U2 : Inport  Port=2
  Change_time : Inport  Port=3
  Abs : Abs  SaturateOnIntegerOverflow=off
  Abs2 : Abs  SaturateOnIntegerOverflow=off
  Add Constant : Bias  Bias=1  SaturateOnIntegerOverflow=off
  Add Constant2 : Bias  Bias=1  SaturateOnIntegerOverflow=off
  Add Constant3 : Bias  Bias=1  SaturateOnIntegerOverflow=off
  Add3 : Sum
  Add4 : Sum  Inputs=+-
  Add5 : Sum
  Clock1 : Clock
  Constant : Constant
  Constant3 : Constant
  Divide : Product  Inputs=/*
  Divide1 : Product  Inputs=**
  Divide4 : Product  Inputs=*/
  Divide5 : Product  Inputs=**
  Divide6 : Product  Inputs=**
  Divide8 : Product  Inputs=*/
  Gain : Gain  Gain=1/2
  Gain1 : Gain  Gain=2
  Gain2 : Gain  Gain=1000
  Gain3 : Gain  Gain=0.001
  Gain5 : Gain  Gain=1/2
  K : Constant  Value=1.5
  Power{,3..5} (4 alike) : Math  Operator=pow
  Reciprocal : Product  Inputs=/
  Reciprocal2 : Product  Inputs=/
  Round1 : Rounding  Operator=round
  Saturation : Saturate  UpperLimit=100  LowerLimit=-100
  Scope : Scope  NumInputPorts=3
  Subtract : Sum  Inputs=+-
  Subtract1 : Sum  Inputs=+-
  Subtract2 : Sum  Inputs=+-
  Sum1 : Sum  Inputs=|-+
  h : Constant  Value=4
  u_out : Outport
  wires:
  Add5/1 -> Scope/1, Saturation/1
  h/1 -> Abs2/1, Divide8/1, Subtract/2
  Add3/1 -> Divide6/2
  Add4/1 -> Divide5/1
  Constant3/1 -> Add3/2, Add4/1
  Power5/1 -> Divide4/2
  Reciprocal2/1 -> Power5/2
  K/1 -> Power4/2, Reciprocal2/1, Reciprocal/1, Power/2
  Gain5/1 -> Divide6/1
  Change_time/1 -> Sum1/1
  Abs/1 -> Power4/1
  Clock1/1 -> Sum1/2
  Gain3/1 -> Subtract/1
  U2/1 -> Gain5/1, Scope/2, Divide1/1
  Round1/1 -> Gain3/1
  Power4/1 -> Add Constant/1
  Gain2/1 -> Round1/1
  Add Constant/1 -> Power5/1
  Subtract/1 -> Divide4/1, Abs/1
  U1/1 -> Subtract2/1, Scope/3
  Divide6/1 -> Add5/1
  Sum1/1 -> Gain2/1  "Elapsed Time"
  Divide4/1 -> Add3/1, Add4/2
  Abs2/1 -> Power/1
  Power/1 -> Add Constant2/1
  Add Constant2/1 -> Power3/1
  Reciprocal/1 -> Power3/2
  Power3/1 -> Divide8/2
  Divide8/1 -> Add Constant3/1
  Add Constant3/1 -> Gain/1
  Constant/1 -> Subtract1/1
  Gain/1 -> Gain1/1, Subtract1/2  "P"
  Subtract1/1 -> Divide1/2
  Divide1/1 -> Subtract2/2
  Subtract2/1 -> Divide/2
  Gain1/1 -> Divide/1
  Divide/1 -> Divide5/2
  Divide5/1 -> Add5/2
  Saturation/1 -> u_out/1

== system CCModel_71/Cruise Control/Version 7.1/Switches ==
  U : Inport
  Throttle_In : Inport  Port=2
  Brake_In : Inport  Port=3
  Add Constant : Bias  Bias=6  SaturateOnIntegerOverflow=off
  Add Constant1 : Bias  Bias=10  SaturateOnIntegerOverflow=off
  Add Constant2 : Bias  Bias=5  SaturateOnIntegerOverflow=off
  Add Constant3 : Bias  Bias=-10  SaturateOnIntegerOverflow=off
  Brake_Switch1 : Switch  Criteria=u2 > Threshold  Threshold=-10  SaturateOnIntegerOverflow=off  InputSameDT=off
  Brake_Switch2 : Switch  Criteria=u2 > Threshold  Threshold=30  SaturateOnIntegerOverflow=off  InputSameDT=off
  Brake_Switch3 : Switch  Criteria=u2 > Threshold  Threshold=5  SaturateOnIntegerOverflow=off  InputSameDT=off
  Constant : Constant  Value=0
  Constant1 : Constant  Value=0
  Gain : Gain  Gain=-1
  Gain1 : Gain  Gain=pi/40
  Gain2 : Gain  Gain=-5
  Gain3 : Gain  Gain=0.2
  Max1 : MinMax  Function=max  Inputs=2
  Polynomial : Polyval  Coefs=[-0.01,0.2,0,0]
  Polynomial1 : Polyval  Coefs=[0.01,0.2,0,10]
  Ramp1 : simulink/Sources/Ramp  slope=5  start=0  InitialOutput=-100
  Saturation1 : Saturate  UpperLimit=100  LowerLimit=-100
  Scope1 : Scope  NumInputPorts=3
  Sin : Trigonometry
  Switch : Switch  Criteria=u2 > Threshold  Threshold=10  SaturateOnIntegerOverflow=off  InputSameDT=off
  Switch1 : Switch  Criteria=u2 > Threshold  Threshold=-20  SaturateOnIntegerOverflow=off  InputSameDT=off
  Throttle_Switch1 : Switch  Criteria=u2 > Threshold  SaturateOnIntegerOverflow=off  InputSameDT=off
  Throttle_Switch3 : Switch  Criteria=u2 > Threshold  Threshold=5  SaturateOnIntegerOverflow=off  InputSameDT=off
  Throttle : Outport
  Brake : Outport  Port=2
  wires:
  Saturation1/1 -> Brake_Switch2/2, Brake_Switch1/2, Switch1/2, Gain/1, Add Constant3/1, Add Constant1/1, Switch/1, Switch/2, Scope1/1, Polynomial/1, Throttle_Switch1/2
  Throttle_Switch1/1 -> Add Constant/1  "Throttle"
  Brake_Switch3/1 -> Scope1/3, Brake/1
  Brake_In/1 -> Brake_Switch3/1, Max1/2
  Throttle_In/1 -> Throttle_Switch3/1, Max1/1
  Throttle_Switch3/1 -> Scope1/2, Throttle/1
  Constant1/1 -> Throttle_Switch1/3, Brake_Switch2/1
  Switch/1 -> Throttle_Switch1/1
  Polynomial/1 -> Switch/3
  Max1/1 -> Throttle_Switch3/2, Brake_Switch3/2
  Add Constant/1 -> Throttle_Switch3/3
  Add Constant1/1 -> Polynomial1/1
  Gain/1 -> Switch1/3
  Polynomial1/1 -> Switch1/1
  Switch1/1 -> Brake_Switch1/3
  Gain1/1 -> Sin/1
  Sin/1 -> Gain2/1
  Gain2/1 -> Add Constant2/1
  Add Constant2/1 -> Brake_Switch1/1
  Brake_Switch2/1 -> Gain3/1  "Brake"
  Brake_Switch1/1 -> Brake_Switch2/3  "Brake"
  U/1 -> Saturation1/1
  Add Constant3/1 -> Gain1/1
  Gain3/1 -> Brake_Switch3/3

== system CCModel_71/Cruise Control/Version 7.2/Apply_Grade ==
  note: This has not been implemented but may be helpful
  note: +(2/5)|P|
  note: x is u, which is linear and g is grade which is sigmoided
  U_in : Inport
  Grade : Inport  Port=2
  Add : Sum
  Add Constant : Bias  Bias=1  SaturateOnIntegerOverflow=off
  Divide : Product  Inputs=*/
  Gain : Gain  Gain=0.8
  Gain1 : Gain  Gain=0.25
  Scope : Scope  NumInputPorts=2
  Sqrt : Sqrt
  Square : Math  Operator=square
  U_Out : Outport
  wires:
  U_in/1 -> Scope/1, Gain/1
  Square/1 -> Add Constant/1
  Add Constant/1 -> Sqrt/1
  Grade/1 -> Gain1/1, Square/1
  Gain1/1 -> Divide/1
  Sqrt/1 -> Divide/2
  Divide/1 -> Add/2
  Gain/1 -> Add/1
  Add/1 -> Scope/2, U_Out/1

== system CCModel_71/Cruise Control/Version 7.2/Detect Change ==
  note: This subsystem detects either a change in the reference velocity, or the driver releasing one of the pedals. It outputs the time of the change, the value of u just before the change, and a boolean "hasChanged" value
  desired_velocity : Inport
  throttle_const : Inport  Port=2
  brake_const : Inport  Port=3
  Smoothed u : Inport  Port=4
  (False) : Constant  Value=0
  (True) : Constant
  AND : Logic  IconShape=distinctive  AllPortsSameDT=off  OutDataTypeStr=boolean
  Clock : Clock
  Delay : Delay  DelayLength=1
  Delay1 : Delay  DelayLength=1
  Detect Change : simulink/Logic and Bit Operations/Detect Change  vinit=0  OutDataTypeStr=boolean
  Detect Change1 : simulink/Logic and Bit Operations/Detect Change  vinit=0  OutDataTypeStr=boolean
  Max : MinMax  Function=max  Inputs=2
  OR : Logic  Operator=OR  IconShape=distinctive  AllPortsSameDT=off  OutDataTypeStr=boolean
  Pedal_threshold : Constant
  Scope : Scope
  Subtract : Sum  Inputs=+-
  Switch : Switch  Criteria=u2 > Threshold  SaturateOnIntegerOverflow=off  InputSameDT=off
  Switch1 : Switch  Criteria=u2 > Threshold  SaturateOnIntegerOverflow=off  InputSameDT=off
  Switch2 : Switch  Criteria=u2 > Threshold  SaturateOnIntegerOverflow=off  InputSameDT=off
  Change_time : Outport
  Old u : Outport  Port=2
  hasChanged : Outport  Port=3
  wires:
  desired_velocity/1 -> Detect Change/1
  Detect Change/1 -> OR/1
  OR/1 -> Switch/2, Switch2/2, hasChanged/1
  Switch1/1 -> Detect Change1/1, Delay1/1
  AND/1 -> OR/2
  Clock/1 -> Switch/1
  Max/1 -> Subtract/1
  (True)/1 -> Switch1/1
  brake_const/1 -> Max/2
  Pedal_threshold/1 -> Subtract/2
  Subtract/1 -> Switch1/2
  (False)/1 -> Switch1/3
  throttle_const/1 -> Max/1
  Delay/1 -> Switch2/1
  Switch/1 -> Switch/3, Scope/1, Change_time/1
  Smoothed u/1 -> Delay/1
  Detect Change1/1 -> AND/2
  Delay1/1 -> AND/1
  Switch2/1 -> Old u/1, Switch2/3

== system CCModel_71/Cruise Control/Version 7.2/PID Controller ==
  note: Typical PID controller, outputs a value between -100 and 100
  error : Inport
  Grade : Inport  Port=2
  Add : Sum
  Add1 : Sum
  Derivative : Derivative
  GKi : Gain  Gain=0
  GKp : Gain  Gain=0
  Integrator : Integrator
  Integrator1 : Integrator
  Kd : Gain  Gain=0.1
  Ki : Gain  Gain=0.03
  Kp : Gain  Gain=4.8
  Saturation : Saturate  Commented=through  UpperLimit=100  LowerLimit=-100
  Scope1 : Scope  NumInputPorts=3
  Sum : Sum  Inputs=+++
  u : Outport
  wires:
  Integrator/1 -> Ki/1
  error/1 -> Integrator/1, Kp/1, Derivative/1  "D"
  Kp/1 -> Scope1/1, Sum/2  "P"
  Ki/1 -> Sum/1, Scope1/2  "I"
  Saturation/1 -> u/1
  Derivative/1 -> Kd/1
  Kd/1 -> Scope1/3, Sum/3  "D"
  Sum/1 -> Add1/1
  Add1/1 -> Saturation/1
  Grade/1 -> Integrator1/1, GKp/1
  Integrator1/1 -> GKi/1
  GKi/1 -> Add/1
  GKp/1 -> Add/2
  Add/1 -> Add1/2

== system CCModel_71/Cruise Control/Version 7.2/Sigmoid ==
  note: This whole part is just to eliminate weird cancellation errors that were happening
  U1 : Inport
  U2 : Inport  Port=2
  Change_time : Inport  Port=3
  hasChanged : Inport  Port=4
  Abs : Abs  SaturateOnIntegerOverflow=off
  Abs2 : Abs  SaturateOnIntegerOverflow=off
  Add Constant : Bias  Bias=1  SaturateOnIntegerOverflow=off
  Add Constant2 : Bias  Bias=1  SaturateOnIntegerOverflow=off
  Add Constant3 : Bias  Bias=1  SaturateOnIntegerOverflow=off
  Add3 : Sum
  Add4 : Sum  Inputs=+-
  Add5 : Sum
  Clock1 : Clock
  Constant : Constant
  Constant3 : Constant
  Divide : Product  Inputs=/*
  Divide1 : Product  Inputs=**
  Divide4 : Product  Inputs=*/
  Divide5 : Product  Inputs=**
  Divide6 : Product  Inputs=**
  Divide8 : Product  Inputs=*/
  Gain : Gain  Gain=1/2
  Gain1 : Gain  Gain=2
  Gain2 : Gain  Gain=1000
  Gain3 : Gain  Gain=0.001
  Gain5 : Gain  Gain=1/2
  K : Constant  Value=1.5
  Power{,3..5} (4 alike) : Math  Operator=pow
  Reciprocal : Product  Inputs=/
  Reciprocal2 : Product  Inputs=/
  Round1 : Rounding  Operator=round
  Saturation : Saturate  UpperLimit=100  LowerLimit=-100
  Scope : Scope  NumInputPorts=3
  Subtract : Sum  Inputs=+-
  Subtract1 : Sum  Inputs=+-
  Subtract2 : Sum  Inputs=+-
  Sum1 : Sum  Inputs=|-+
  h : Constant  Value=4
  u_out : Outport
  wires:
  Add5/1 -> Saturation/1, Scope/2  "Smoothed"
  h/1 -> Abs2/1, Divide8/1, Subtract/2
  Add3/1 -> Divide6/2
  Add4/1 -> Divide5/1
  Constant3/1 -> Add3/2, Add4/1
  Power5/1 -> Divide4/2
  Reciprocal2/1 -> Power5/2
  K/1 -> Power4/2, Reciprocal2/1, Reciprocal/1, Power/2
  Gain5/1 -> Divide6/1
  Change_time/1 -> Sum1/1
  Abs/1 -> Power4/1
  Clock1/1 -> Sum1/2
  Gain3/1 -> Subtract/1
  U2/1 -> Scope/1, Gain5/1, Divide1/1
  Round1/1 -> Gain3/1
  Power4/1 -> Add Constant/1
  Gain2/1 -> Round1/1
  Add Constant/1 -> Power5/1
  Subtract/1 -> Divide4/1, Abs/1
  U1/1 -> Scope/3, Subtract2/1
  Divide6/1 -> Add5/1
  Sum1/1 -> Gain2/1  "Elapsed Time"
  Divide4/1 -> Add3/1, Add4/2
  Abs2/1 -> Power/1
  Power/1 -> Add Constant2/1
  Add Constant2/1 -> Power3/1
  Reciprocal/1 -> Power3/2
  Power3/1 -> Divide8/2
  Divide8/1 -> Add Constant3/1
  Add Constant3/1 -> Gain/1
  Constant/1 -> Subtract1/1
  Gain/1 -> Gain1/1, Subtract1/2  "P"
  Subtract1/1 -> Divide1/2
  Divide1/1 -> Subtract2/2
  Subtract2/1 -> Divide/2
  Gain1/1 -> Divide/1
  Divide/1 -> Divide5/2
  Divide5/1 -> Add5/2
  Saturation/1 -> u_out/1

== system CCModel_71/Cruise Control/Version 7.2/Switches ==
  U : Inport
  Throttle_In : Inport  Port=2
  Brake_In : Inport  Port=3
  Add Constant : Bias  Bias=6  SaturateOnIntegerOverflow=off
  Brake_Switch1 : Switch  Criteria=u2 > Threshold  Threshold=30  SaturateOnIntegerOverflow=off  InputSameDT=off
  Brake_Switch3 : Switch  Criteria=u2 > Threshold  Threshold=5  SaturateOnIntegerOverflow=off  InputSameDT=off
  Constant : Constant  Value=0
  Constant1 : Constant  Value=0
  Gain : Gain  Gain=-1
  Gain3 : Gain  Gain=0.2
  Max1 : MinMax  Function=max  Inputs=2
  Polynomial : Polyval  Coefs=[-0.01,0.2,0,0]
  Polynomial1 : Polyval  Coefs=[6.66666666666666666666666666666666666e-7,-9.33333333333333333333333333333333e-05,0.0105,-0.448,6]
  Ramp1 : simulink/Sources/Ramp  slope=5  start=0  InitialOutput=-100
  Saturation1 : Saturate  UpperLimit=100  LowerLimit=-100
  Scope1 : Scope  NumInputPorts=3
  Switch : Switch  Criteria=u2 > Threshold  Threshold=10  SaturateOnIntegerOverflow=off  InputSameDT=off
  Switch1 : Switch  Criteria=u2 > Threshold  Threshold=-20  SaturateOnIntegerOverflow=off  InputSameDT=off
  Throttle_Switch1 : Switch  Criteria=u2 > Threshold  SaturateOnIntegerOverflow=off  InputSameDT=off
  Throttle_Switch3 : Switch  Criteria=u2 > Threshold  Threshold=5  SaturateOnIntegerOverflow=off  InputSameDT=off
  Throttle : Outport
  Brake : Outport  Port=2
  wires:
  Throttle_Switch1/1 -> Add Constant/1  "Throttle"
  Brake_Switch3/1 -> Scope1/3, Brake/1
  Brake_In/1 -> Brake_Switch3/1, Max1/2
  Throttle_In/1 -> Throttle_Switch3/1, Max1/1
  Throttle_Switch3/1 -> Scope1/2, Throttle/1
  Constant1/1 -> Brake_Switch1/1, Throttle_Switch1/3
  Switch/1 -> Throttle_Switch1/1
  Polynomial/1 -> Switch/3
  Max1/1 -> Throttle_Switch3/2, Brake_Switch3/2
  Add Constant/1 -> Throttle_Switch3/3
  Saturation1/1 -> Polynomial1/1, Brake_Switch1/2, Switch1/2, Gain/1, Switch/1, Switch/2, Scope1/1, Polynomial/1, Throttle_Switch1/2
  Gain/1 -> Switch1/3
  Polynomial1/1 -> Switch1/1
  Switch1/1 -> Brake_Switch1/3
  Brake_Switch1/1 -> Gain3/1  "Brake"
  Gain3/1 -> Brake_Switch3/3
  U/1 -> Saturation1/1

== system CCModel_71/Cruise Control/Version 7.3/Apply_Grade ==
  U_in : Inport
  Grade : Inport  Port=2
  Add : Sum
  Add Constant : Bias  Bias=1  SaturateOnIntegerOverflow=off
  Divide : Product  Inputs=*/
  Gain : Gain  Gain=0.8
  Gain1 : Gain  Gain=0.3
  Sqrt : Sqrt
  Square : Math  Operator=square
  U_Out : Outport
  wires:
  U_in/1 -> Gain/1
  Square/1 -> Add Constant/1
  Add Constant/1 -> Sqrt/1
  Grade/1 -> Gain1/1, Square/1
  Gain1/1 -> Divide/1
  Sqrt/1 -> Divide/2
  Divide/1 -> Add/2
  Gain/1 -> Add/1
  Add/1 -> U_Out/1

== system CCModel_71/Cruise Control/Version 7.3/Detect Change ==
  desired_velocity : Inport
  throttle_const : Inport  Port=2
  brake_const : Inport  Port=3
  Smoothed u : Inport  Port=4
  error : Inport  Port=5
  (False) : Constant  Value=0
  (True) : Constant
  AND : Logic  IconShape=distinctive  AllPortsSameDT=off  OutDataTypeStr=boolean
  Abs : Abs  SaturateOnIntegerOverflow=off
  Change_Desired_Speed : Subsystem
  Clock : Clock
  Constant : Constant
  Constant1 : Constant  Value=0
  Delay : Delay  DelayLength=1
  Delay1 : Delay  DelayLength=1
  Detect Change : simulink/Logic and Bit Operations/Detect Change  vinit=0  OutDataTypeStr=boolean
  Detect Change1 : simulink/Logic and Bit Operations/Detect Change  vinit=0  OutDataTypeStr=boolean
  Driver Control : Subsystem
  Error_Equal_Zero : Subsystem
  Max : MinMax  Function=max  Inputs=2
  OR : Logic  Operator=OR  IconShape=distinctive  AllPortsSameDT=off  OutDataTypeStr=boolean
  OR1 : Logic  Operator=OR  IconShape=distinctive  AllPortsSameDT=off  OutDataTypeStr=boolean
  Pedal_threshold : Constant  Value=5
  Subtract : Sum  Inputs=+-
  Switch : Switch  Criteria=u2 > Threshold  SaturateOnIntegerOverflow=off  InputSameDT=off
  Switch1 : Switch  Criteria=u2 > Threshold  SaturateOnIntegerOverflow=off  InputSameDT=off
  Switch2 : Switch  Criteria=u2 > Threshold  SaturateOnIntegerOverflow=off  InputSameDT=off
  Switch3 : Switch  Criteria=u2 > Threshold  Threshold=0.01  SaturateOnIntegerOverflow=off  InputSameDT=off
  Change_time : Outport
  Old u : Outport  Port=2
  hasChanged : Outport  Port=3
  ChangeTrigger : Outport  Port=4
  wires:
  desired_velocity/1 -> Detect Change/1
  Detect Change/1 -> OR/1
  OR/1 -> OR1/2, ChangeTrigger/1
  Switch1/1 -> Detect Change1/1, Delay1/1
  AND/1 -> OR/2
  Clock/1 -> Switch/1
  Max/1 -> Subtract/1
  (True)/1 -> Switch1/1
  brake_const/1 -> Max/2
  Pedal_threshold/1 -> Subtract/2
  Subtract/1 -> Switch1/2
  (False)/1 -> Switch1/3
  throttle_const/1 -> Max/1
  Delay/1 -> Switch2/1
  Switch/1 -> Switch/3, Change_time/1
  Smoothed u/1 -> Delay/1
  Detect Change1/1 -> AND/2
  Delay1/1 -> AND/1
  Switch2/1 -> Old u/1, Switch2/3
  error/1 -> Abs/1  "D"
  Constant/1 -> Switch3/3
  Abs/1 -> Switch3/2
  Constant1/1 -> Switch3/1
  Switch3/1 -> OR1/1
  OR1/1 -> Switch2/2, Switch/2, hasChanged/1
